simulink model "gm_whdlOFDMTx"  (R2022b)
settings: Solver=FixedStepDiscrete  StartTime=0.0  StopTime=0  RelTol=1e-3
model workspace (MATLAB code in the model file):
  | config = whdlexamples.OFDMTxParameters();
  | fftLen = config.fftLen;
  | subC = config.subC;
  | cpLen = config.cpLen;
  | fs = config.fs;
  | NSS = config.NSS;
  | NRS = config.NRS;
  | NHeader = config.NHeader;
  | NData = config.NData;
  | NSymPerF = config.NSymPerF;
  | ssSymbol = config.ssSymbol;
  | rsSymbol = config.rsSymbol;
  | NHeaderBits = config.NHeaderBits;
  | headerCRCBool = config.headerCRCBool;
  | headerConvK = config.headerConvK;
  | headerConvCode = config.headerConvCode;
  | pilotValPerSym = config.pilotValPerSym;
  | pilotLen = config.pilotLen;
  | dataCRCPoly = config.dataCRCPoly;
  | dataCRCBool = config.dataCRCBool;
  | dataCRCLen = config.dataCRCLen;
  | dataConvK = config.dataConvK;
  | dataConvCode = config.dataConvCode;
  | scramInit = config.scramInit;
  | firCoeff = config.firCoeff;
  | rateFac1 = config.rateFac1;
  | rateFac2 = config.rateFac2;
  | headerLat = config.headerLat;
  | headerTime = config.headerTime;
  | preambleInd = config.preambleInd;
  | headerDataInd = config.headerDataInd;
  | trBlkSize = config.trBlkSize;
  | randOFDM = config.randOFDM;
  | headerIntrlvMaxBlkSize = config.headerIntrlvMaxBlkSize;
  | headerIntrlvNColumns   = config.headerIntrlvNColumns;
  | dataIntrlvMaxBlkSize   = config.dataIntrlvMaxBlkSize;
  | dataIntrlvNColumns     = config.dataIntrlvNColumns;
  | clear config
libraries: hdlsllib x49, simulink x22, dspsigops x11, whdlmod x3, whdledac x3, whdlutilities x2, commhdlcrc x2, dsphdlfiltering2 x1
(part 4 of 4)

== matlab function gm_whdlOFDMTx/Frame Generator/Header/Header Formation/Header Formation ==
  data: modType input; headerBits output; codeRate input; fftLen input; validIn input; startOut output; endOut output; validOut output; NHeaderBits parameter
function [headerBits,startOut,endOut,validOut]= formHeader(modType,codeRate,fftLen,validIn,NHeaderBits)
%#codegen
% This function takes fftLen, modType and codeRate inputs to form Header Bits
% NHeaderBits is the total number of Header Bits formed

persistent modReg codeReg fftReg validReg startInt startO endO validO count countReg buffer1 buffer2 map

if(isempty(modReg))
    modReg   = fi(0,0,2,0);
    codeReg  = fi(0,0,2,0);
    fftReg   = fi(0,0,3,0);
    validReg = false;
    startInt = false;
    startO   = false(2,1);
    endO     = false;
    validO   = false(2,1);
    count    = fi(1,0,nextpow2(NHeaderBits),0);
    countReg = fi([1 1],0,nextpow2(NHeaderBits),0);
    buffer1  = false(NHeaderBits,1);
    buffer2  = false(NHeaderBits,1);  
    map      = logical([0   0   0;...       % Header Bits are formed from                
                        0   0   1;...       % 'map', based on inputs
                        0   1   0;...
                        0   1   1;...
                        1   0   0;...
                        1   0   1;...
                        1   1   0;...
                        1   1   1]');
end
             

% Assign outputs
headerBits = buffer2(countReg(2));
startOut   = startO(2);
endOut     = endO;
validOut   = validO(2);
   
% Generate start, end control signals    
endO = (count(:) == NHeaderBits);  
if(startInt)
    if(count(:) == NHeaderBits)
        startInt = false;
        count(:) = 1;
    else
        count(:) = count+1;
    end
end
startO(2)   = startO(1);
validO(2)   = validO(1);
buffer2     = buffer1;
countReg(2) = countReg(1);

% Form Header bits based on stored register values and generate valid signal
if(validReg)
    count(:)       = 1;
    startInt       = true;
    buffer1(1:3)   = map(1:3,fftReg+1);       % Form 3 fftBits based on 'fftLen' input
    buffer1(4:5)   = map(2:3,modReg+1);       % Form 2 modBits based on 'modType' input
    buffer1(6:7)   = map(2:3,codeReg+1);      % Form 2 codeBits based on 'codeRate' input
    buffer1(8:end) = false(NHeaderBits-7,1);  % Append 15 nullBits available for future use
end
startO(1)   = validReg;
validO(1)   = startInt;
countReg(1) = count;

% Store inputs in registers
modReg(:)  = modType;
codeReg(:) = codeRate;
fftReg(:)  = fftLen;
validReg   = validIn;
end
